simulink model "ex2"  (R2020a)
settings: Solver=VariableStepAuto  StartTime=0.0  StopTime=10.0  RelTol=1e-3

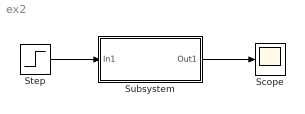
== system ex2 ==
  Scope : Scope
  Step : Step  SampleTime=0
  Subsystem : Subsystem  mask{C=10000, R=0.0001}
      mask prompts: C "C="; R "R="
  wires:
  Step/1 -> Subsystem/1(In1)
  Subsystem/1(Out1) -> Scope/1

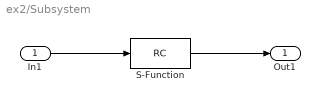
== system ex2/Subsystem ==
  In1 : Inport
  S-Function : S-Function  FunctionName=RC  Parameters=A,B,C  SFunctionDeploymentMode=off  EnableBusSupport=off  mask{A=-1/(R*C), B=1/(R*C), C=1}
      mask prompts: A "A="; B "B="; C "C="
  Out1 : Outport
  wires:
  In1/1 -> S-Function/1
  S-Function/1 -> Out1/1
